simulink model "W01_Base_World_point_cloud_performance_cs"  (R2019a)
settings: Solver=FixedStepDiscrete  StartTime=0.0  StopTime=612  FixedStep=1/20  RelTol=1e-3
PreLoadFcn:
  | mbxruntime.callbacks.PreLoadFcn(bdroot);
  | check_NUTS_defined
  | model_closed = 0;
  | assignin('base',['model_closed_' bdroot],false);
PostLoadFcn:
  | mbxruntime.callbacks.PostLoadFcn(bdroot);
InitFcn:
  | mbxruntime.callbacks.InitFcn(bdroot);
StartFcn:
  | mbxruntime.callbacks.StartFcn(bdroot);
StopFcn:
  | mbxruntime.callbacks.StopFcn(bdroot);;
  | 
model workspace: external: MAT-File .\W01_Base_World_point_cloud_performance_cs_hws.mat (data not in the file)
undefined symbols (not defined in the file or in its folder): DiscIntNeverNeededParam, mbxruntime, Orientation, Position, tabledata, W01_Base_World_point_cloud_performance_cs_040d40f1a6998015, W01_Base_World_point_cloud_performance_cs_1139c7b998f0a907, W01_Base_World_point_cloud_performance_cs_282394bd9d11aaf9, W01_Base_World_point_cloud_performance_cs_287b60bdf29e1a5e, W01_Base_World_point_cloud_performance_cs_3d871abdbcb86cf3, W01_Base_World_point_cloud_performance_cs_8fcb18657fabefaa, W01_Base_World_point_cloud_performance_cs_9753c0e86959d2d1, W01_Base_World_point_cloud_performance_cs_9a36d3aa72057750, W01_Base_World_point_cloud_performance_cs_9a6e020116cabe98, W01_Base_World_point_cloud_performance_cs_a4ac4280946ec032, W01_Base_World_point_cloud_performance_cs_bbd2f0877d622aa1, W01_Base_World_point_cloud_performance_cs_d5d898f74cbe8316, W01_Base_World_point_cloud_performance_cs_d7d451946b8970f9, W01_Base_World_point_cloud_performance_cs_ed2f0fc632b9c889, W01_Base_World_point_cloud_performance_cs_f0849590441458e2, W01_Base_World_point_cloud_performance_cs_fc0d0ecba8ca3fae
libraries: simulink_extras x30, simulink x10, adeye_lib x6, sharedtransform x2, robotlib x2
(part 2 of 8)

== system W01_Base_World_point_cloud_performance_cs/ANIM_Child_RegularAni_1 ==
  ANIM_Child_RegularAni_1 : Inport  Tag=inport/AnimationOutport  OutDataTypeStr=Bus: PRESCAN_ANIMACTUATORDATA  PortDimensions=1  SampleTime=1/20  BusOutputAsStruct=on
  Actuator : S-Function  FunctionName=sfun_AnimActuator  Parameters=mbxruntime.parameters.convert(UniqueID), mbxruntime.parameters.convert(TimeStep)  SFunctionDeploymentMode=off  EnableBusSupport=off  mask(PreScan Sink Block: State Animation){UniqueID=18395, TimeStep=1/20}
      mask prompts: UniqueID "Auto-Assigned: Unique ID"; TimeStep "Auto-Assigned: Upload Period [s]"
      mask help: The Human Animation port allows the human to walk, run or bend
      mask Help: eval('openHelp(239)')
      mask Display: image(imread('HumanAnimated.jpg'))
  wires:
  ANIM_Child_RegularAni_1/1 -> Actuator/1

== system W01_Base_World_point_cloud_performance_cs/ANIM_Child_RegularAni_2 ==
  ANIM_Child_RegularAni_2 : Inport  Tag=inport/AnimationOutport  OutDataTypeStr=Bus: PRESCAN_ANIMACTUATORDATA  PortDimensions=1  SampleTime=1/20  BusOutputAsStruct=on
  Actuator : S-Function  FunctionName=sfun_AnimActuator  Parameters=mbxruntime.parameters.convert(UniqueID), mbxruntime.parameters.convert(TimeStep)  SFunctionDeploymentMode=off  EnableBusSupport=off  mask(PreScan Sink Block: State Animation){UniqueID=18628, TimeStep=1/20}
      mask prompts: UniqueID "Auto-Assigned: Unique ID"; TimeStep "Auto-Assigned: Upload Period [s]"
      mask help: The Human Animation port allows the human to walk, run or bend
      mask Help: eval('openHelp(239)')
      mask Display: image(imread('HumanAnimated.jpg'))
  wires:
  ANIM_Child_RegularAni_2/1 -> Actuator/1

== system W01_Base_World_point_cloud_performance_cs/ANIM_Female_RegularAni_1 ==
  ANIM_Female_RegularAni_1 : Inport  Tag=inport/AnimationOutport  OutDataTypeStr=Bus: PRESCAN_ANIMACTUATORDATA  PortDimensions=1  SampleTime=1/20  BusOutputAsStruct=on
  Actuator : S-Function  FunctionName=sfun_AnimActuator  Parameters=mbxruntime.parameters.convert(UniqueID), mbxruntime.parameters.convert(TimeStep)  SFunctionDeploymentMode=off  EnableBusSupport=off  mask(PreScan Sink Block: State Animation){UniqueID=18631, TimeStep=1/20}
      mask prompts: UniqueID "Auto-Assigned: Unique ID"; TimeStep "Auto-Assigned: Upload Period [s]"
      mask help: The Human Animation port allows the human to walk, run or bend
      mask Help: eval('openHelp(239)')
      mask Display: image(imread('HumanAnimated.jpg'))
  wires:
  ANIM_Female_RegularAni_1/1 -> Actuator/1

== system W01_Base_World_point_cloud_performance_cs/ANIM_Male_RegularAni_1 ==
  ANIM_Male_RegularAni_1 : Inport  Tag=inport/AnimationOutport  OutDataTypeStr=Bus: PRESCAN_ANIMACTUATORDATA  PortDimensions=1  SampleTime=1/20  BusOutputAsStruct=on
  Actuator : S-Function  FunctionName=sfun_AnimActuator  Parameters=mbxruntime.parameters.convert(UniqueID), mbxruntime.parameters.convert(TimeStep)  SFunctionDeploymentMode=off  EnableBusSupport=off  mask(PreScan Sink Block: State Animation){UniqueID=18634, TimeStep=1/20}
      mask prompts: UniqueID "Auto-Assigned: Unique ID"; TimeStep "Auto-Assigned: Upload Period [s]"
      mask help: The Human Animation port allows the human to walk, run or bend
      mask Help: eval('openHelp(239)')
      mask Display: image(imread('HumanAnimated.jpg'))
  wires:
  ANIM_Male_RegularAni_1/1 -> Actuator/1

== system W01_Base_World_point_cloud_performance_cs/ANIM_Male_RegularAni_2 ==
  ANIM_Male_RegularAni_2 : Inport  Tag=inport/AnimationOutport  OutDataTypeStr=Bus: PRESCAN_ANIMACTUATORDATA  PortDimensions=1  SampleTime=1/20  BusOutputAsStruct=on
  Actuator : S-Function  FunctionName=sfun_AnimActuator  Parameters=mbxruntime.parameters.convert(UniqueID), mbxruntime.parameters.convert(TimeStep)  SFunctionDeploymentMode=off  EnableBusSupport=off  mask(PreScan Sink Block: State Animation){UniqueID=18853, TimeStep=1/20}
      mask prompts: UniqueID "Auto-Assigned: Unique ID"; TimeStep "Auto-Assigned: Upload Period [s]"
      mask help: The Human Animation port allows the human to walk, run or bend
      mask Help: eval('openHelp(239)')
      mask Display: image(imread('HumanAnimated.jpg'))
  wires:
  ANIM_Male_RegularAni_2/1 -> Actuator/1

== system W01_Base_World_point_cloud_performance_cs/Audi_A8_Sedan_1 ==
  SELF_Audi_A8_Sedan_1 : Inport  Tag=inport/SelfPort  OutDataTypeStr=Bus: PRESCAN_SELFSENSORDATA  PortDimensions=1  SampleTime=1/20  BusOutputAsStruct=on
  Car_Pos_and_Orient : Subsystem
  Path : S-Function  LoadFcn=load('PrescanMotionData.mat')  FunctionName=sfun_Path  Parameters=mbxruntime.parameters.convert(uniqueID), pathUniqueID, mbxruntime.parameters.convert(timestep)  SFunctionDeploymentMode=off  EnableBusSupport=off  mask(Path){uniqueID=18645, pathUniqueID=W01_Base_World_point_cloud_performance_cs_f0849590441458e2, timestep=1/20}
      mask prompts: uniqueID "Object Unique ID"; pathUniqueID "Path Unique ID"; timestep "MATLAB timestep:"
      mask help:
      | The path block outputs the position along a given trajectory.
      |
      | For more information, please click Help.
      mask Help: eval('openHelp(312)')
      mask Display: image(imread('Path.png'))
  SELF_Demux : Subsystem  Tag=demux/SelfPort  mask(PreScan Demux Block:){}
      mask help:
      | The SELF port shows (state) information of the actor itself. The outputs are position in the experiment's axis system and the GPS coordinates, and the object's absolute velocity and compass heading.
      |
      | For more information, please click Help.
      settings: DeleteFcn=PreScanBlockDeleteFcn;
      mask Help: eval('openHelp(462)')
      mask Display:
      | port_label('output',1,'x [m]')
      | port_label('output',2,'y [m]')
      | port_label('output',3,'z [m]','texmode','on')
      | port_label('output',4,'Rotx [deg]','texmode','on')
      | port_label('output',5,'Roty [deg]','texmode','on')
      | port_label('output',6,'Rotz [deg]','texmode','on')
      | port_label('output',7,'GPS lat [deg]','texmode','on')
      | port_label('output',8,'GPS long [deg]','texmode','on')
      | port_label('output',9,'GPS alt [m]','texmode','on')
      | port_label('output',10,'Velocity [m/s]')
      | port_label('output',11,'Heading [deg]')
      | port_label('output',12,'Yaw rate [deg/s]')
      | port_label('output',13,'Timestamp [s]')
  STATE_Audi_A8_Sedan_1_rc : RateTransition  Tag=mux_rc/StatePort  OutPortSampleTimeOpt=Inherit
  SpeedProfile : S-Function  LoadFcn=load('PrescanMotionData.mat')  FunctionName=sfun_SpeedProfile  Parameters=speedProfileUniqueID, mbxruntime.parameters.convert(timestep)  SFunctionDeploymentMode=off  EnableBusSupport=off  mask(SpeedProfile){speedProfileUniqueID=W01_Base_World_point_cloud_performance_cs_a4ac4280946ec032, timestep=1/20}
      mask prompts: speedProfileUniqueID "Speed Profile Unique ID"; timestep "MATLAB timestep:"
      mask help:
      | The speed profile block outputs the travelled distance, velocities and acceleration along a given path.
      |
      | For more information, please click Help.
      mask Help: eval('openHelp(312)')
      mask Display: image(imread('SpeedProfile.png'))
  Terminator_{1..7} (7 alike) : Terminator
  message_creator : Subsystem
  STATE_Audi_A8_Sedan_1_bus : Outport  Tag=outport/StatePort  OutDataTypeStr=Bus: PRESCAN_STATEACTUATORDATA  PortDimensions=1  SampleTime=1/20
  SafetyPlannerLoc : Outport  Port=2
  wires:
  Car_Pos_and_Orient/1(Out1) -> message_creator/1(In1)
  message_creator/1(Out1) -> SafetyPlannerLoc/1
  SELF_Demux/1(x [m]) -> Car_Pos_and_Orient/1(In1)
  SELF_Demux/2(y [m]) -> Car_Pos_and_Orient/2(In2)
  SELF_Demux/3(z [m]) -> Car_Pos_and_Orient/3(In3)
  SELF_Demux/4(rotx [deg]) -> Car_Pos_and_Orient/4(In4)
  SELF_Demux/5(roty [deg]) -> Car_Pos_and_Orient/5(In5)
  SELF_Demux/6(rotz [deg]) -> Car_Pos_and_Orient/6(In6)
  STATE_Audi_A8_Sedan_1_rc/1 -> STATE_Audi_A8_Sedan_1_bus/1
  SpeedProfile/1 -> Path/1
  Path/1 -> STATE_Audi_A8_Sedan_1_rc/1
  SELF_Audi_A8_Sedan_1/1 -> SELF_Demux/1(SELF)
  SELF_Demux/7(GPS lat [deg]) -> Terminator_1/1
  SELF_Demux/8(GPS long [deg]) -> Terminator_2/1
  SELF_Demux/9(GPS alt [m]) -> Terminator_3/1
  SELF_Demux/10(velocity [m/s]) -> Terminator_4/1
  SELF_Demux/11(heading [deg]) -> Terminator_5/1
  SELF_Demux/12(yaw rate [deg/s]) -> Terminator_6/1
  SELF_Demux/13(TimeStamp [s]) -> Terminator_7/1

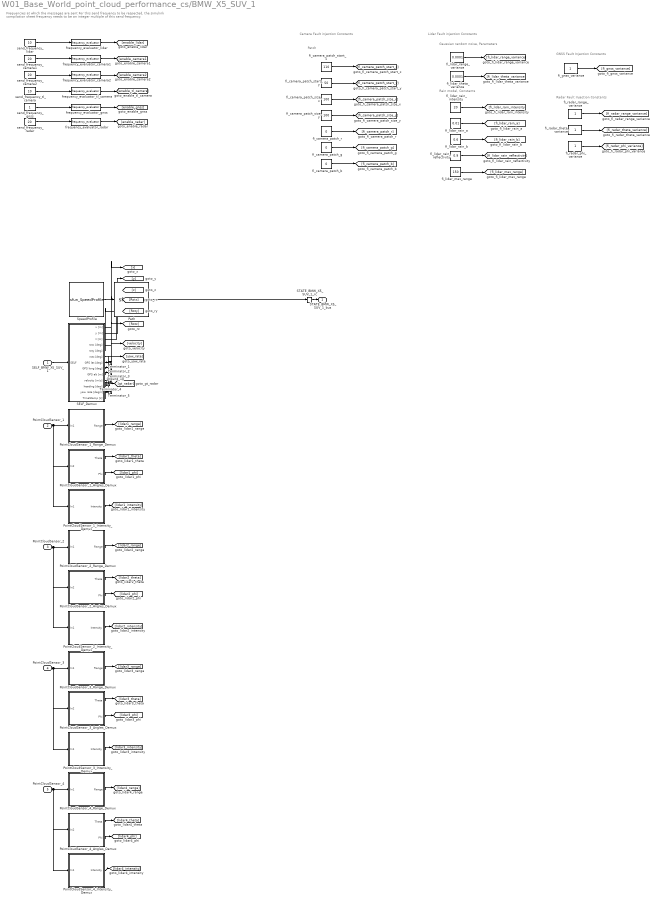
== system W01_Base_World_point_cloud_performance_cs/BMW_X5_SUV_1 ==
  note: Frequencies at which the messages are sent
      |
      | For this send frequency to be respected, the simulink compilation sheet frequency
      | needs to be an integer multiple of this send frequency.
  note: Lidar Fault injection Constants
  note: Camera Fault injection Constants
  note: Patch
  note: Rain model, Constants
  note: Radar Fault Injection Constants
  note: Gaussian random noise, Parameters
  note: GNSS Fault Injection Constants
  SELF_BMW_X5_SUV_1 : Inport  Tag=inport/SelfPort  OutDataTypeStr=Bus: PRESCAN_SELFSENSORDATA  PortDimensions=1  SampleTime=1/20  BusOutputAsStruct=on
  PointCloudSensor_1 : Inport  Tag=inport/PointCloudInport  Port=2  OutDataTypeStr=single  SampleTime=1/10  BusOutputAsStruct=on
  PointCloudSensor_2 : Inport  Tag=inport/PointCloudInport  Port=3  OutDataTypeStr=single  SampleTime=1/10  BusOutputAsStruct=on
  PointCloudSensor_3 : Inport  Tag=inport/PointCloudInport  Port=4  OutDataTypeStr=single  SampleTime=1/10  BusOutputAsStruct=on
  PointCloudSensor_4 : Inport  Tag=inport/PointCloudInport  Port=5  OutDataTypeStr=single  SampleTime=1/10  BusOutputAsStruct=on
  Ground_10 : Ground
  Path : S-Function  LoadFcn=load('PrescanMotionData.mat')  FunctionName=sfun_Path  Parameters=mbxruntime.parameters.convert(uniqueID), pathUniqueID, mbxruntime.parameters.convert(timestep)  SFunctionDeploymentMode=off  EnableBusSupport=off  mask(Path){uniqueID=9040, pathUniqueID=W01_Base_World_point_cloud_performance_cs_9a36d3aa72057750, timestep=1/20}
      mask prompts: uniqueID "Object Unique ID"; pathUniqueID "Path Unique ID"; timestep "MATLAB timestep:"
      mask help:
      | The path block outputs the position along a given trajectory.
      |
      | For more information, please click Help.
      mask Help: eval('openHelp(312)')
      mask Display: image(imread('Path.png'))
  PointCloudSensor_1_Angles_Demux : Subsystem  Tag=demux/PCS/Angles  mask{SensorName=PointCloudSensor_1, offset=225, hres=225, vres=16}
      mask prompts: SensorName "Sensor Name"; offset "Data Start"; hres "Horizontal Resolution"; vres "Vertical Resolution"
      mask Help: eval('openHelp(6400)')
      mask Display:
      | fprintf('Point Cloud:\n Data\n %s \n %d x %d px',SensorName,hres,vres)
      | port_label('output',1,'Theta')
      | port_label('output',2,'Phi')
  PointCloudSensor_1_Intensity_Demux : Subsystem  Tag=demux/PCS/Intensity  mask{SensorName=PointCloudSensor_1, offset=675, hres=225, vres=16}
      mask prompts: SensorName "Sensor Name"; offset "Data Start"; hres "Horizontal Resolution"; vres "Vertical Resolution"
      mask Help: eval('openHelp(6400)')
      mask Display:
      | fprintf('Point Cloud:\n Data\n %s \n %d x %d px',SensorName,hres,vres)
      | port_label('output',1,'Intensity')
  PointCloudSensor_1_Range_Demux : Subsystem  Tag=demux/PCS/Range  mask{SensorName=PointCloudSensor_1, offset=0, hres=225, vres=16}
      mask prompts: SensorName "Sensor Name"; offset "Data Start"; hres "Horizontal Resolution"; vres "Vertical Resolution"
      mask Help: eval('openHelp(6400)')
      mask Display:
      | fprintf('Point Cloud:\n Data\n %s \n %d x %d px',SensorName,hres,vres)
      | port_label('output',1,'Range')
  PointCloudSensor_2_Angles_Demux : Subsystem  Tag=demux/PCS/Angles  mask{SensorName=PointCloudSensor_2, offset=225, hres=225, vres=16}
      mask prompts: SensorName "Sensor Name"; offset "Data Start"; hres "Horizontal Resolution"; vres "Vertical Resolution"
      mask Help: eval('openHelp(6400)')
      mask Display:
      | fprintf('Point Cloud:\n Data\n %s \n %d x %d px',SensorName,hres,vres)
      | port_label('output',1,'Theta')
      | port_label('output',2,'Phi')
  PointCloudSensor_2_Intensity_Demux : Subsystem  Tag=demux/PCS/Intensity  mask{SensorName=PointCloudSensor_2, offset=675, hres=225, vres=16}
      mask prompts: SensorName "Sensor Name"; offset "Data Start"; hres "Horizontal Resolution"; vres "Vertical Resolution"
      mask Help: eval('openHelp(6400)')
      mask Display:
      | fprintf('Point Cloud:\n Data\n %s \n %d x %d px',SensorName,hres,vres)
      | port_label('output',1,'Intensity')
  PointCloudSensor_2_Range_Demux : Subsystem  Tag=demux/PCS/Range  mask{SensorName=PointCloudSensor_2, offset=0, hres=225, vres=16}
      mask prompts: SensorName "Sensor Name"; offset "Data Start"; hres "Horizontal Resolution"; vres "Vertical Resolution"
      mask Help: eval('openHelp(6400)')
      mask Display:
      | fprintf('Point Cloud:\n Data\n %s \n %d x %d px',SensorName,hres,vres)
      | port_label('output',1,'Range')
  PointCloudSensor_3_Angles_Demux : Subsystem  Tag=demux/PCS/Angles  mask{SensorName=PointCloudSensor_3, offset=225, hres=225, vres=16}
      mask prompts: SensorName "Sensor Name"; offset "Data Start"; hres "Horizontal Resolution"; vres "Vertical Resolution"
      mask Help: eval('openHelp(6400)')
      mask Display:
      | fprintf('Point Cloud:\n Data\n %s \n %d x %d px',SensorName,hres,vres)
      | port_label('output',1,'Theta')
      | port_label('output',2,'Phi')
  PointCloudSensor_3_Intensity_Demux : Subsystem  Tag=demux/PCS/Intensity  mask{SensorName=PointCloudSensor_3, offset=675, hres=225, vres=16}
      mask prompts: SensorName "Sensor Name"; offset "Data Start"; hres "Horizontal Resolution"; vres "Vertical Resolution"
      mask Help: eval('openHelp(6400)')
      mask Display:
      | fprintf('Point Cloud:\n Data\n %s \n %d x %d px',SensorName,hres,vres)
      | port_label('output',1,'Intensity')
  PointCloudSensor_3_Range_Demux : Subsystem  Tag=demux/PCS/Range  mask{SensorName=PointCloudSensor_3, offset=0, hres=225, vres=16}
      mask prompts: SensorName "Sensor Name"; offset "Data Start"; hres "Horizontal Resolution"; vres "Vertical Resolution"
      mask Help: eval('openHelp(6400)')
      mask Display:
      | fprintf('Point Cloud:\n Data\n %s \n %d x %d px',SensorName,hres,vres)
      | port_label('output',1,'Range')
  PointCloudSensor_4_Angles_Demux : Subsystem  Tag=demux/PCS/Angles  mask{SensorName=PointCloudSensor_4, offset=225, hres=225, vres=16}
      mask prompts: SensorName "Sensor Name"; offset "Data Start"; hres "Horizontal Resolution"; vres "Vertical Resolution"
      mask Help: eval('openHelp(6400)')
      mask Display:
      | fprintf('Point Cloud:\n Data\n %s \n %d x %d px',SensorName,hres,vres)
      | port_label('output',1,'Theta')
      | port_label('output',2,'Phi')
  PointCloudSensor_4_Intensity_Demux : Subsystem  Tag=demux/PCS/Intensity  mask{SensorName=PointCloudSensor_4, offset=675, hres=225, vres=16}
      mask prompts: SensorName "Sensor Name"; offset "Data Start"; hres "Horizontal Resolution"; vres "Vertical Resolution"
      mask Help: eval('openHelp(6400)')
      mask Display:
      | fprintf('Point Cloud:\n Data\n %s \n %d x %d px',SensorName,hres,vres)
      | port_label('output',1,'Intensity')
  PointCloudSensor_4_Range_Demux : Subsystem  Tag=demux/PCS/Range  mask{SensorName=PointCloudSensor_4, offset=0, hres=225, vres=16}
      mask prompts: SensorName "Sensor Name"; offset "Data Start"; hres "Horizontal Resolution"; vres "Vertical Resolution"
      mask Help: eval('openHelp(6400)')
      mask Display:
      | fprintf('Point Cloud:\n Data\n %s \n %d x %d px',SensorName,hres,vres)
      | port_label('output',1,'Range')
  SELF_Demux : Subsystem  Tag=demux/SelfPort  mask(PreScan Demux Block:){}
      mask help:
      | The SELF port shows (state) information of the actor itself. The outputs are position in the experiment's axis system and the GPS coordinates, and the object's absolute velocity and compass heading.
      |
      | For more information, please click Help.
      settings: DeleteFcn=PreScanBlockDeleteFcn;
      mask Help: eval('openHelp(462)')
      mask Display:
      | port_label('output',1,'x [m]')
      | port_label('output',2,'y [m]')
      | port_label('output',3,'z [m]','texmode','on')
      | port_label('output',4,'Rotx [deg]','texmode','on')
      | port_label('output',5,'Roty [deg]','texmode','on')
      | port_label('output',6,'Rotz [deg]','texmode','on')
      | port_label('output',7,'GPS lat [deg]','texmode','on')
      | port_label('output',8,'GPS long [deg]','texmode','on')
      | port_label('output',9,'GPS alt [m]','texmode','on')
      | port_label('output',10,'Velocity [m/s]')
      | port_label('output',11,'Heading [deg]')
      | port_label('output',12,'Yaw rate [deg/s]')
      | port_label('output',13,'Timestamp [s]')
  STATE_BMW_X5_SUV_1_rc : RateTransition  Tag=mux_rc/StatePort  OutPortSampleTimeOpt=Inherit
  SpeedProfile : S-Function  LoadFcn=load('PrescanMotionData.mat')  FunctionName=sfun_SpeedProfile  Parameters=speedProfileUniqueID, mbxruntime.parameters.convert(timestep)  SFunctionDeploymentMode=off  EnableBusSupport=off  mask(SpeedProfile){speedProfileUniqueID=W01_Base_World_point_cloud_performance_cs_9753c0e86959d2d1, timestep=1/20}
      mask prompts: speedProfileUniqueID "Speed Profile Unique ID"; timestep "MATLAB timestep:"
      mask help:
      | The speed profile block outputs the travelled distance, velocities and acceleration along a given path.
      |
      | For more information, please click Help.
      mask Help: eval('openHelp(312)')
      mask Display: image(imread('SpeedProfile.png'))
  Terminator_{1..5} (5 alike) : Terminator
  fi_camera_patch_b : Constant  Value=0
  fi_camera_patch_g : Constant  Value=0
  fi_camera_patch_r : Constant  Value=0
  fi_camera_patch_size_x : Constant  Value=100
  fi_camera_patch_size_y : Constant  Value=100
  fi_camera_patch_start_x : Constant  Value=110
  fi_camera_patch_start_y : Constant  Value=50
  fi_gnss_variance : Constant
  fi_lidar_max_range : Constant  Value=150
  fi_lidar_rain_a : Constant  Value=0.01
  fi_lidar_rain_b : Constant  Value=0.6
  fi_lidar_rain_intensity : Constant  Value=20
  fi_lidar_rain_reflectivity : Constant  Value=0.9
  fi_lidar_range_variance : Constant  Value=0.0001
  fi_lidar_theta_variance : Constant  Value=0.0001
  fi_radar_phi_variance : Constant
  fi_radar_range_variance : Constant
  fi_radar_theta_variance : Constant
  frequency_evaluator_camera1 : adeye_lib/frequency_evaluator  SystemSampleTime=-1
  frequency_evaluator_camera2 : adeye_lib/frequency_evaluator  SystemSampleTime=-1
  frequency_evaluator_gnss : adeye_lib/frequency_evaluator  SystemSampleTime=-1
  frequency_evaluator_lidar : adeye_lib/frequency_evaluator  SystemSampleTime=-1
      link override Constant: Value=0.999
  frequency_evaluator_radar : adeye_lib/frequency_evaluator  SystemSampleTime=-1
  frequency_evaluator_tl_camera : adeye_lib/frequency_evaluator  SystemSampleTime=-1
  send_frequency_camera1 : Constant  Value=20
  send_frequency_camera2 : Constant  Value=20
  send_frequency_gnss : Constant
  send_frequency_lidar : Constant  Value=10
  send_frequency_radar : Constant  Value=20
  send_frequency_tl_camera : Constant  Value=10
  STATE_BMW_X5_SUV_1_bus : Outport  Tag=outport/StatePort  OutDataTypeStr=Bus: PRESCAN_STATEACTUATORDATA  PortDimensions=1  SampleTime=1/20
  wires:
  fi_camera_patch_b/1 -> [fi_camera_patch_b]
  fi_camera_patch_g/1 -> [fi_camera_patch_g]
  fi_camera_patch_r/1 -> [fi_camera_patch_r]
  fi_camera_patch_size_x/1 -> [fi_camera_patch_size_x]
  fi_camera_patch_size_y/1 -> [fi_camera_patch_size_y]
  fi_camera_patch_start_x/1 -> [fi_camera_patch_start_x]
  fi_camera_patch_start_y/1 -> [fi_camera_patch_start_y]
  fi_gnss_variance/1 -> [fi_gnss_variance]
  fi_lidar_max_range/1 -> [fi_lidar_max_range]
  fi_lidar_rain_a/1 -> [fi_lidar_rain_a]
  fi_lidar_rain_b/1 -> [fi_lidar_rain_b]
  fi_lidar_rain_intensity/1 -> [fi_lidar_rain_intensity]
  fi_lidar_rain_reflectivity/1 -> [fi_lidar_rain_reflectivity]
  fi_lidar_range_variance/1 -> [fi_lidar_range_variance]
  fi_lidar_theta_variance/1 -> [fi_lidar_theta_variance]
  fi_radar_phi_variance/1 -> [fi_radar_phi_variance]
  fi_radar_range_variance/1 -> [fi_radar_range_variance]
  fi_radar_theta_variance/1 -> [fi_radar_theta_variance]
  PointCloudSensor_1_Intensity_Demux/1(Intensity) -> [lidar1_intensity]
  PointCloudSensor_1_Angles_Demux/2(Phi) -> [lidar1_phi]
  PointCloudSensor_1_Range_Demux/1(Range) -> [lidar1_range]
  PointCloudSensor_1_Angles_Demux/1(Theta) -> [lidar1_theta]
  PointCloudSensor_2_Intensity_Demux/1(Intensity) -> [lidar2_intensity]
  PointCloudSensor_2_Angles_Demux/2(Phi) -> [lidar2_phi]
  PointCloudSensor_2_Range_Demux/1(Range) -> [lidar2_range]
  PointCloudSensor_2_Angles_Demux/1(Theta) -> [lidar2_theta]
  PointCloudSensor_3_Intensity_Demux/1(Intensity) -> [lidar3_intensity]
  PointCloudSensor_3_Angles_Demux/2(Phi) -> [lidar3_phi]
  PointCloudSensor_3_Range_Demux/1(Range) -> [lidar3_range]
  PointCloudSensor_3_Angles_Demux/1(Theta) -> [lidar3_theta]
  PointCloudSensor_4_Intensity_Demux/1(Intensity) -> [lidar4_intensity]
  PointCloudSensor_4_Angles_Demux/2(Phi) -> [lidar4_phi]
  PointCloudSensor_4_Range_Demux/1(Range) -> [lidar4_range]
  PointCloudSensor_4_Angles_Demux/1(Theta) -> [lidar4_theta]
  SELF_Demux/4(rotx [deg]) -> [Rotx]
  SELF_Demux/5(roty [deg]) -> [Roty]
  SELF_Demux/6(rotz [deg]) -> [Rotz]
  SELF_Demux/10(velocity [m/s]) -> [velocity]
  SELF_Demux/1(x [m]) -> [x]
  SELF_Demux/2(y [m]) -> [y]
  SELF_Demux/12(yaw rate [deg/s]) -> [yaw_rate]
  SELF_Demux/3(z [m]) -> [z]
  send_frequency_lidar/1 -> frequency_evaluator_lidar/1
  send_frequency_camera1/1 -> frequency_evaluator_camera1/1
  send_frequency_camera2/1 -> frequency_evaluator_camera2/1
  send_frequency_tl_camera/1 -> frequency_evaluator_tl_camera/1
  send_frequency_gnss/1 -> frequency_evaluator_gnss/1
  frequency_evaluator_lidar/1 -> [enable_lidar]
  frequency_evaluator_camera1/1 -> [enable_camera1]
  frequency_evaluator_camera2/1 -> [enable_camera2]
  frequency_evaluator_tl_camera/1 -> [enable_tl_camera]
  frequency_evaluator_gnss/1 -> [enable_gnss]
  send_frequency_radar/1 -> frequency_evaluator_radar/1
  frequency_evaluator_radar/1 -> [enable_radar]
  STATE_BMW_X5_SUV_1_rc/1 -> STATE_BMW_X5_SUV_1_bus/1
  SpeedProfile/1 -> Path/1
  Path/1 -> STATE_BMW_X5_SUV_1_rc/1
  SELF_BMW_X5_SUV_1/1 -> SELF_Demux/1(SELF)
  PointCloudSensor_1/1 -> PointCloudSensor_1_Range_Demux/1(In1), PointCloudSensor_1_Angles_Demux/1(In2), PointCloudSensor_1_Intensity_Demux/1(In1)
  PointCloudSensor_2/1 -> PointCloudSensor_2_Range_Demux/1(In1), PointCloudSensor_2_Angles_Demux/1(In2), PointCloudSensor_2_Intensity_Demux/1(In1)
  PointCloudSensor_3/1 -> PointCloudSensor_3_Range_Demux/1(In1), PointCloudSensor_3_Angles_Demux/1(In2), PointCloudSensor_3_Intensity_Demux/1(In1)
  PointCloudSensor_4/1 -> PointCloudSensor_4_Range_Demux/1(In1), PointCloudSensor_4_Angles_Demux/1(In2), PointCloudSensor_4_Intensity_Demux/1(In1)
  SELF_Demux/7(GPS lat [deg]) -> Terminator_1/1
  SELF_Demux/8(GPS long [deg]) -> Terminator_2/1
  SELF_Demux/9(GPS alt [m]) -> Terminator_3/1
  SELF_Demux/11(heading [deg]) -> Terminator_4/1
  SELF_Demux/13(TimeStamp [s]) -> Terminator_5/1
  Ground_10/1 -> [gt_radar]

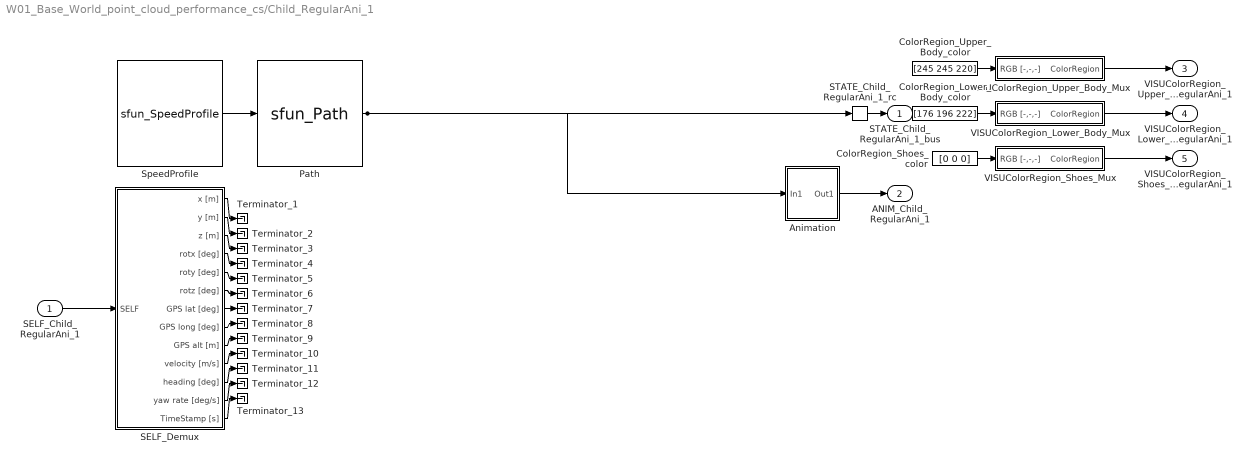
== system W01_Base_World_point_cloud_performance_cs/Child_RegularAni_1 ==
  SELF_Child_RegularAni_1 : Inport  Tag=inport/SelfPort  OutDataTypeStr=Bus: PRESCAN_SELFSENSORDATA  PortDimensions=1  SampleTime=1/20  BusOutputAsStruct=on
  Animation : Subsystem  Tag=RunningHumanAnimation  mask(Prescan Conversion Block: Running Human Animation){MWS=1.95, WalkingScale=1.0, RunningScale=1.0, TimeStep=1/20}
      mask prompts: MWS "Maximum Walking Speed [m/s], above which the animation will switch to running mode."; WalkingScale "Walking mode scaling factor to sync the animation frames to the displacement."; RunningScale "Running mode scaling factor to sync the animation frames to the displacement."; TimeStep "Auto-Assigned: Upload Period [s]"
      mask help: The Running Human Animation block converts the State signal of a human into signals to properly control the animation.
      mask Help: eval('openHelp(239)');
      mask Display: image(imread('HumanAnimated.jpg'))
  ColorRegion_Lower_Body_color : Constant  Tag=VisuLightConst  Value=[176 196 222]
  ColorRegion_Shoes_color : Constant  Tag=VisuLightConst  Value=[0 0 0]
  ColorRegion_Upper_Body_color : Constant  Tag=VisuLightConst  Value=[245 245 220]
  Path : S-Function  LoadFcn=load('PrescanMotionData.mat')  FunctionName=sfun_Path  Parameters=mbxruntime.parameters.convert(uniqueID), pathUniqueID, mbxruntime.parameters.convert(timestep)  SFunctionDeploymentMode=off  EnableBusSupport=off  mask(Path){uniqueID=18395, pathUniqueID=W01_Base_World_point_cloud_performance_cs_d7d451946b8970f9, timestep=1/20}
      mask prompts: uniqueID "Object Unique ID"; pathUniqueID "Path Unique ID"; timestep "MATLAB timestep:"
      mask help:
      | The path block outputs the position along a given trajectory.
      |
      | For more information, please click Help.
      mask Help: eval('openHelp(312)')
      mask Display: image(imread('Path.png'))
  SELF_Demux : Subsystem  Tag=demux/SelfPort  mask(PreScan Demux Block:){}
      mask help:
      | The SELF port shows (state) information of the actor itself. The outputs are position in the experiment's axis system and the GPS coordinates, and the object's absolute velocity and compass heading.
      |
      | For more information, please click Help.
      settings: DeleteFcn=PreScanBlockDeleteFcn;
      mask Help: eval('openHelp(462)')
      mask Display:
      | port_label('output',1,'x [m]')
      | port_label('output',2,'y [m]')
      | port_label('output',3,'z [m]','texmode','on')
      | port_label('output',4,'Rotx [deg]','texmode','on')
      | port_label('output',5,'Roty [deg]','texmode','on')
      | port_label('output',6,'Rotz [deg]','texmode','on')
      | port_label('output',7,'GPS lat [deg]','texmode','on')
      | port_label('output',8,'GPS long [deg]','texmode','on')
      | port_label('output',9,'GPS alt [m]','texmode','on')
      | port_label('output',10,'Velocity [m/s]')
      | port_label('output',11,'Heading [deg]')
      | port_label('output',12,'Yaw rate [deg/s]')
      | port_label('output',13,'Timestamp [s]')
  STATE_Child_RegularAni_1_rc : RateTransition  Tag=mux_rc/StatePort  OutPortSampleTimeOpt=Inherit
  SpeedProfile : S-Function  LoadFcn=load('PrescanMotionData.mat')  FunctionName=sfun_SpeedProfile  Parameters=speedProfileUniqueID, mbxruntime.parameters.convert(timestep)  SFunctionDeploymentMode=off  EnableBusSupport=off  mask(SpeedProfile){speedProfileUniqueID=W01_Base_World_point_cloud_performance_cs_bbd2f0877d622aa1, timestep=1/20}
      mask prompts: speedProfileUniqueID "Speed Profile Unique ID"; timestep "MATLAB timestep:"
      mask help:
      | The speed profile block outputs the travelled distance, velocities and acceleration along a given path.
      |
      | For more information, please click Help.
      mask Help: eval('openHelp(312)')
      mask Display: image(imread('SpeedProfile.png'))
  Terminator_{1..13} (13 alike) : Terminator
  VISUColorRegion_Lower_Body_Mux : Subsystem  Tag=mux/MuxColorRegion  LoadFcn=load PrescanColorData  mask(PreScan User Interface: VisuTextureColor){}
      mask help:
      | The VisuTextureColor block provides a way to adapt the color of a vehicle.
      |
      | For more information, please click Help.
      settings: DeleteFcn=PreScanBlockDeleteFcn;
      mask Help: eval('openHelp(230)')
  VISUColorRegion_Shoes_Mux : Subsystem  Tag=mux/MuxColorRegion  LoadFcn=load PrescanColorData  mask(PreScan User Interface: VisuTextureColor){}
      mask help:
      | The VisuTextureColor block provides a way to adapt the color of a vehicle.
      |
      | For more information, please click Help.
      settings: DeleteFcn=PreScanBlockDeleteFcn;
      mask Help: eval('openHelp(230)')
  VISUColorRegion_Upper_Body_Mux : Subsystem  Tag=mux/MuxColorRegion  LoadFcn=load PrescanColorData  mask(PreScan User Interface: VisuTextureColor){}
      mask help:
      | The VisuTextureColor block provides a way to adapt the color of a vehicle.
      |
      | For more information, please click Help.
      settings: DeleteFcn=PreScanBlockDeleteFcn;
      mask Help: eval('openHelp(230)')
  STATE_Child_RegularAni_1_bus : Outport  Tag=outport/StatePort  OutDataTypeStr=Bus: PRESCAN_STATEACTUATORDATA  PortDimensions=1  SampleTime=1/20
  ANIM_Child_RegularAni_1 : Outport  Tag=outport/AnimationOutport  Port=2  OutDataTypeStr=Bus: PRESCAN_ANIMACTUATORDATA  PortDimensions=1  SampleTime=1/20
  VISUColorRegion_Upper_Body_Child_RegularAni_1 : Outport  Tag=outport/ColorRegion  Port=3  OutDataTypeStr=Bus: PRESCAN_COLOR_DATA  PortDimensions=1  SampleTime=1/20
  VISUColorRegion_Lower_Body_Child_RegularAni_1 : Outport  Tag=outport/ColorRegion  Port=4  OutDataTypeStr=Bus: PRESCAN_COLOR_DATA  PortDimensions=1  SampleTime=1/20
  VISUColorRegion_Shoes_Child_RegularAni_1 : Outport  Tag=outport/ColorRegion  Port=5  OutDataTypeStr=Bus: PRESCAN_COLOR_DATA  PortDimensions=1  SampleTime=1/20
  wires:
  STATE_Child_RegularAni_1_rc/1 -> STATE_Child_RegularAni_1_bus/1
  Animation/1(Out1) -> ANIM_Child_RegularAni_1/1
  SpeedProfile/1 -> Path/1
  Path/1 -> STATE_Child_RegularAni_1_rc/1, Animation/1(In1)
  SELF_Child_RegularAni_1/1 -> SELF_Demux/1(SELF)
  VISUColorRegion_Upper_Body_Mux/1(ColorRegion) -> VISUColorRegion_Upper_Body_Child_RegularAni_1/1
  ColorRegion_Upper_Body_color/1 -> VISUColorRegion_Upper_Body_Mux/1(RGB [-,-,-])
  VISUColorRegion_Lower_Body_Mux/1(ColorRegion) -> VISUColorRegion_Lower_Body_Child_RegularAni_1/1
  ColorRegion_Lower_Body_color/1 -> VISUColorRegion_Lower_Body_Mux/1(RGB [-,-,-])
  VISUColorRegion_Shoes_Mux/1(ColorRegion) -> VISUColorRegion_Shoes_Child_RegularAni_1/1
  ColorRegion_Shoes_color/1 -> VISUColorRegion_Shoes_Mux/1(RGB [-,-,-])
  SELF_Demux/1(x [m]) -> Terminator_1/1
  SELF_Demux/2(y [m]) -> Terminator_2/1
  SELF_Demux/3(z [m]) -> Terminator_3/1
  SELF_Demux/4(rotx [deg]) -> Terminator_4/1
  SELF_Demux/5(roty [deg]) -> Terminator_5/1
  SELF_Demux/6(rotz [deg]) -> Terminator_6/1
  SELF_Demux/7(GPS lat [deg]) -> Terminator_7/1
  SELF_Demux/8(GPS long [deg]) -> Terminator_8/1
  SELF_Demux/9(GPS alt [m]) -> Terminator_9/1
  SELF_Demux/10(velocity [m/s]) -> Terminator_10/1
  SELF_Demux/11(heading [deg]) -> Terminator_11/1
  SELF_Demux/12(yaw rate [deg/s]) -> Terminator_12/1
  SELF_Demux/13(TimeStamp [s]) -> Terminator_13/1

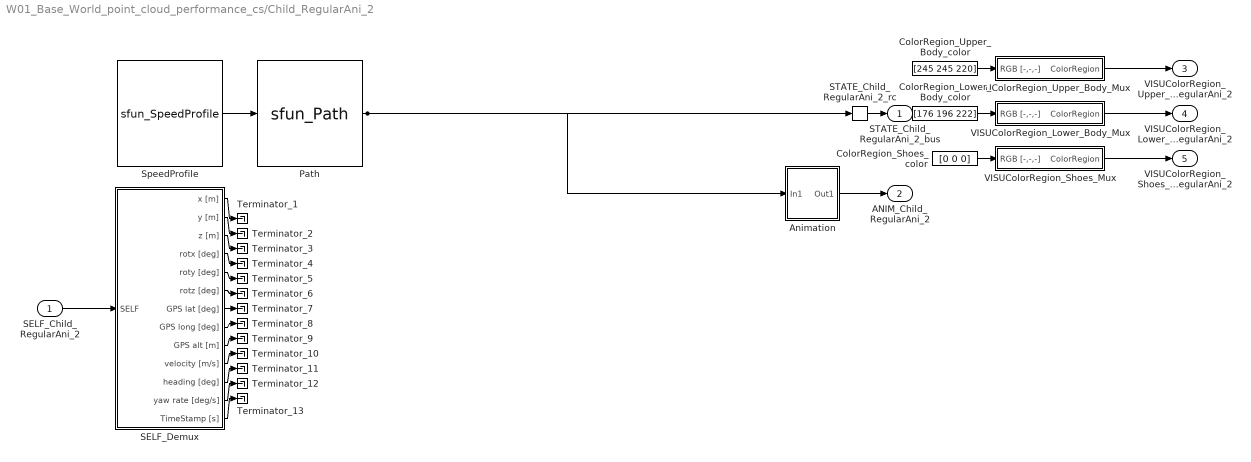
== system W01_Base_World_point_cloud_performance_cs/Child_RegularAni_2 ==
  SELF_Child_RegularAni_2 : Inport  Tag=inport/SelfPort  OutDataTypeStr=Bus: PRESCAN_SELFSENSORDATA  PortDimensions=1  SampleTime=1/20  BusOutputAsStruct=on
  Animation : Subsystem  Tag=RunningHumanAnimation  mask(Prescan Conversion Block: Running Human Animation){MWS=1.95, WalkingScale=1.0, RunningScale=1.0, TimeStep=1/20}
      mask prompts: MWS "Maximum Walking Speed [m/s], above which the animation will switch to running mode."; WalkingScale "Walking mode scaling factor to sync the animation frames to the displacement."; RunningScale "Running mode scaling factor to sync the animation frames to the displacement."; TimeStep "Auto-Assigned: Upload Period [s]"
      mask help: The Running Human Animation block converts the State signal of a human into signals to properly control the animation.
      mask Help: eval('openHelp(239)');
      mask Display: image(imread('HumanAnimated.jpg'))
  ColorRegion_Lower_Body_color : Constant  Tag=VisuLightConst  Value=[176 196 222]
  ColorRegion_Shoes_color : Constant  Tag=VisuLightConst  Value=[0 0 0]
  ColorRegion_Upper_Body_color : Constant  Tag=VisuLightConst  Value=[245 245 220]
  Path : S-Function  LoadFcn=load('PrescanMotionData.mat')  FunctionName=sfun_Path  Parameters=mbxruntime.parameters.convert(uniqueID), pathUniqueID, mbxruntime.parameters.convert(timestep)  SFunctionDeploymentMode=off  EnableBusSupport=off  mask(Path){uniqueID=18628, pathUniqueID=W01_Base_World_point_cloud_performance_cs_d5d898f74cbe8316, timestep=1/20}
      mask prompts: uniqueID "Object Unique ID"; pathUniqueID "Path Unique ID"; timestep "MATLAB timestep:"
      mask help:
      | The path block outputs the position along a given trajectory.
      |
      | For more information, please click Help.
      mask Help: eval('openHelp(312)')
      mask Display: image(imread('Path.png'))
  SELF_Demux : Subsystem  Tag=demux/SelfPort  mask(PreScan Demux Block:){}
      mask help:
      | The SELF port shows (state) information of the actor itself. The outputs are position in the experiment's axis system and the GPS coordinates, and the object's absolute velocity and compass heading.
      |
      | For more information, please click Help.
      settings: DeleteFcn=PreScanBlockDeleteFcn;
      mask Help: eval('openHelp(462)')
      mask Display:
      | port_label('output',1,'x [m]')
      | port_label('output',2,'y [m]')
      | port_label('output',3,'z [m]','texmode','on')
      | port_label('output',4,'Rotx [deg]','texmode','on')
      | port_label('output',5,'Roty [deg]','texmode','on')
      | port_label('output',6,'Rotz [deg]','texmode','on')
      | port_label('output',7,'GPS lat [deg]','texmode','on')
      | port_label('output',8,'GPS long [deg]','texmode','on')
      | port_label('output',9,'GPS alt [m]','texmode','on')
      | port_label('output',10,'Velocity [m/s]')
      | port_label('output',11,'Heading [deg]')
      | port_label('output',12,'Yaw rate [deg/s]')
      | port_label('output',13,'Timestamp [s]')
  STATE_Child_RegularAni_2_rc : RateTransition  Tag=mux_rc/StatePort  OutPortSampleTimeOpt=Inherit
  SpeedProfile : S-Function  LoadFcn=load('PrescanMotionData.mat')  FunctionName=sfun_SpeedProfile  Parameters=speedProfileUniqueID, mbxruntime.parameters.convert(timestep)  SFunctionDeploymentMode=off  EnableBusSupport=off  mask(SpeedProfile){speedProfileUniqueID=W01_Base_World_point_cloud_performance_cs_040d40f1a6998015, timestep=1/20}
      mask prompts: speedProfileUniqueID "Speed Profile Unique ID"; timestep "MATLAB timestep:"
      mask help:
      | The speed profile block outputs the travelled distance, velocities and acceleration along a given path.
      |
      | For more information, please click Help.
      mask Help: eval('openHelp(312)')
      mask Display: image(imread('SpeedProfile.png'))
  Terminator_{1..13} (13 alike) : Terminator
  VISUColorRegion_Lower_Body_Mux : Subsystem  Tag=mux/MuxColorRegion  LoadFcn=load PrescanColorData  mask(PreScan User Interface: VisuTextureColor){}
      mask help:
      | The VisuTextureColor block provides a way to adapt the color of a vehicle.
      |
      | For more information, please click Help.
      settings: DeleteFcn=PreScanBlockDeleteFcn;
      mask Help: eval('openHelp(230)')
  VISUColorRegion_Shoes_Mux : Subsystem  Tag=mux/MuxColorRegion  LoadFcn=load PrescanColorData  mask(PreScan User Interface: VisuTextureColor){}
      mask help:
      | The VisuTextureColor block provides a way to adapt the color of a vehicle.
      |
      | For more information, please click Help.
      settings: DeleteFcn=PreScanBlockDeleteFcn;
      mask Help: eval('openHelp(230)')
  VISUColorRegion_Upper_Body_Mux : Subsystem  Tag=mux/MuxColorRegion  LoadFcn=load PrescanColorData  mask(PreScan User Interface: VisuTextureColor){}
      mask help:
      | The VisuTextureColor block provides a way to adapt the color of a vehicle.
      |
      | For more information, please click Help.
      settings: DeleteFcn=PreScanBlockDeleteFcn;
      mask Help: eval('openHelp(230)')
  STATE_Child_RegularAni_2_bus : Outport  Tag=outport/StatePort  OutDataTypeStr=Bus: PRESCAN_STATEACTUATORDATA  PortDimensions=1  SampleTime=1/20
  ANIM_Child_RegularAni_2 : Outport  Tag=outport/AnimationOutport  Port=2  OutDataTypeStr=Bus: PRESCAN_ANIMACTUATORDATA  PortDimensions=1  SampleTime=1/20
  VISUColorRegion_Upper_Body_Child_RegularAni_2 : Outport  Tag=outport/ColorRegion  Port=3  OutDataTypeStr=Bus: PRESCAN_COLOR_DATA  PortDimensions=1  SampleTime=1/20
  VISUColorRegion_Lower_Body_Child_RegularAni_2 : Outport  Tag=outport/ColorRegion  Port=4  OutDataTypeStr=Bus: PRESCAN_COLOR_DATA  PortDimensions=1  SampleTime=1/20
  VISUColorRegion_Shoes_Child_RegularAni_2 : Outport  Tag=outport/ColorRegion  Port=5  OutDataTypeStr=Bus: PRESCAN_COLOR_DATA  PortDimensions=1  SampleTime=1/20
  wires:
  STATE_Child_RegularAni_2_rc/1 -> STATE_Child_RegularAni_2_bus/1
  Animation/1(Out1) -> ANIM_Child_RegularAni_2/1
  SpeedProfile/1 -> Path/1
  Path/1 -> STATE_Child_RegularAni_2_rc/1, Animation/1(In1)
  SELF_Child_RegularAni_2/1 -> SELF_Demux/1(SELF)
  VISUColorRegion_Upper_Body_Mux/1(ColorRegion) -> VISUColorRegion_Upper_Body_Child_RegularAni_2/1
  ColorRegion_Upper_Body_color/1 -> VISUColorRegion_Upper_Body_Mux/1(RGB [-,-,-])
  VISUColorRegion_Lower_Body_Mux/1(ColorRegion) -> VISUColorRegion_Lower_Body_Child_RegularAni_2/1
  ColorRegion_Lower_Body_color/1 -> VISUColorRegion_Lower_Body_Mux/1(RGB [-,-,-])
  VISUColorRegion_Shoes_Mux/1(ColorRegion) -> VISUColorRegion_Shoes_Child_RegularAni_2/1
  ColorRegion_Shoes_color/1 -> VISUColorRegion_Shoes_Mux/1(RGB [-,-,-])
  SELF_Demux/1(x [m]) -> Terminator_1/1
  SELF_Demux/2(y [m]) -> Terminator_2/1
  SELF_Demux/3(z [m]) -> Terminator_3/1
  SELF_Demux/4(rotx [deg]) -> Terminator_4/1
  SELF_Demux/5(roty [deg]) -> Terminator_5/1
  SELF_Demux/6(rotz [deg]) -> Terminator_6/1
  SELF_Demux/7(GPS lat [deg]) -> Terminator_7/1
  SELF_Demux/8(GPS long [deg]) -> Terminator_8/1
  SELF_Demux/9(GPS alt [m]) -> Terminator_9/1
  SELF_Demux/10(velocity [m/s]) -> Terminator_10/1
  SELF_Demux/11(heading [deg]) -> Terminator_11/1
  SELF_Demux/12(yaw rate [deg/s]) -> Terminator_12/1
  SELF_Demux/13(TimeStamp [s]) -> Terminator_13/1

== system W01_Base_World_point_cloud_performance_cs/Citroen_C3_Hatchback_1 ==
  SELF_Citroen_C3_Hatchback_1 : Inport  Tag=inport/SelfPort  OutDataTypeStr=Bus: PRESCAN_SELFSENSORDATA  PortDimensions=1  SampleTime=1/20  BusOutputAsStruct=on
  Car_Pos_and_Orient : Subsystem
  Path : S-Function  LoadFcn=load('PrescanMotionData.mat')  FunctionName=sfun_Path  Parameters=mbxruntime.parameters.convert(uniqueID), pathUniqueID, mbxruntime.parameters.convert(timestep)  SFunctionDeploymentMode=off  EnableBusSupport=off  mask(Path){uniqueID=18857, pathUniqueID=W01_Base_World_point_cloud_performance_cs_282394bd9d11aaf9, timestep=1/20}
      mask prompts: uniqueID "Object Unique ID"; pathUniqueID "Path Unique ID"; timestep "MATLAB timestep:"
      mask help:
      | The path block outputs the position along a given trajectory.
      |
      | For more information, please click Help.
      mask Help: eval('openHelp(312)')
      mask Display: image(imread('Path.png'))
  SELF_Demux : Subsystem  Tag=demux/SelfPort  mask(PreScan Demux Block:){}
      mask help:
      | The SELF port shows (state) information of the actor itself. The outputs are position in the experiment's axis system and the GPS coordinates, and the object's absolute velocity and compass heading.
      |
      | For more information, please click Help.
      settings: DeleteFcn=PreScanBlockDeleteFcn;
      mask Help: eval('openHelp(462)')
      mask Display:
      | port_label('output',1,'x [m]')
      | port_label('output',2,'y [m]')
      | port_label('output',3,'z [m]','texmode','on')
      | port_label('output',4,'Rotx [deg]','texmode','on')
      | port_label('output',5,'Roty [deg]','texmode','on')
      | port_label('output',6,'Rotz [deg]','texmode','on')
      | port_label('output',7,'GPS lat [deg]','texmode','on')
      | port_label('output',8,'GPS long [deg]','texmode','on')
      | port_label('output',9,'GPS alt [m]','texmode','on')
      | port_label('output',10,'Velocity [m/s]')
      | port_label('output',11,'Heading [deg]')
      | port_label('output',12,'Yaw rate [deg/s]')
      | port_label('output',13,'Timestamp [s]')
  STATE_Citroen_C3_Hatchback_1_rc : RateTransition  Tag=mux_rc/StatePort  OutPortSampleTimeOpt=Inherit
  SpeedProfile : S-Function  LoadFcn=load('PrescanMotionData.mat')  FunctionName=sfun_SpeedProfile  Parameters=speedProfileUniqueID, mbxruntime.parameters.convert(timestep)  SFunctionDeploymentMode=off  EnableBusSupport=off  mask(SpeedProfile){speedProfileUniqueID=W01_Base_World_point_cloud_performance_cs_9a6e020116cabe98, timestep=1/20}
      mask prompts: speedProfileUniqueID "Speed Profile Unique ID"; timestep "MATLAB timestep:"
      mask help:
      | The speed profile block outputs the travelled distance, velocities and acceleration along a given path.
      |
      | For more information, please click Help.
      mask Help: eval('openHelp(312)')
      mask Display: image(imread('SpeedProfile.png'))
  Terminator_{1..7} (7 alike) : Terminator
  message_creator : Subsystem
  STATE_Citroen_C3_Hatchback_1_bus : Outport  Tag=outport/StatePort  OutDataTypeStr=Bus: PRESCAN_STATEACTUATORDATA  PortDimensions=1  SampleTime=1/20
  SafetyPlannerLoc : Outport  Port=2
  wires:
  Car_Pos_and_Orient/1(Out1) -> message_creator/1(In1)
  message_creator/1(Out1) -> SafetyPlannerLoc/1
  SELF_Demux/1(x [m]) -> Car_Pos_and_Orient/1(In1)
  SELF_Demux/2(y [m]) -> Car_Pos_and_Orient/2(In2)
  SELF_Demux/3(z [m]) -> Car_Pos_and_Orient/3(In3)
  SELF_Demux/4(rotx [deg]) -> Car_Pos_and_Orient/4(In4)
  SELF_Demux/5(roty [deg]) -> Car_Pos_and_Orient/5(In5)
  SELF_Demux/6(rotz [deg]) -> Car_Pos_and_Orient/6(In6)
  STATE_Citroen_C3_Hatchback_1_rc/1 -> STATE_Citroen_C3_Hatchback_1_bus/1
  SpeedProfile/1 -> Path/1
  Path/1 -> STATE_Citroen_C3_Hatchback_1_rc/1
  SELF_Citroen_C3_Hatchback_1/1 -> SELF_Demux/1(SELF)
  SELF_Demux/7(GPS lat [deg]) -> Terminator_1/1
  SELF_Demux/8(GPS long [deg]) -> Terminator_2/1
  SELF_Demux/9(GPS alt [m]) -> Terminator_3/1
  SELF_Demux/10(velocity [m/s]) -> Terminator_4/1
  SELF_Demux/11(heading [deg]) -> Terminator_5/1
  SELF_Demux/12(yaw rate [deg/s]) -> Terminator_6/1
  SELF_Demux/13(TimeStamp [s]) -> Terminator_7/1

== system W01_Base_World_point_cloud_performance_cs/Controller ==
  Terminator : Terminator
  sfun_Controller : S-Function  FunctionName=sfun_Controller  Parameters=SParameter1, SParameter2, SParameter3, SParameter4, SParameter5, SParameter6, SParameter7, SParameter8, SParameter9, SParameter10, SampleTime  SFunctionDeploymentMode=off  EnableBusSupport=off  mask(Legacy Function){SFunctionSpec=void prescan_outputFcn(void** work1, PRESCAN_CONTROLLERDATA y1[1]), SParameter1=uint8([ExperimentFile 0]), SParameter2=uint8([ModelDepo 0]), SParameter3=uint8([ControllerOptions 0]), SParameter4=RTmode, SParameter5=PreScanExecutionMode, SParameter6=ControlMode, SParameter7=ControllerCount, SParameter8=ControllerIndex, SParameter9=uint8([SimulationMode 0]), SParameter10=uint8([TargetName 0]), SampleTime=TimeStep, ShowSpec=on}
      mask prompts: SParameter1 "P1:"; SParameter2 "P2:"; SParameter3 "P3:"; SParameter4 "P4:"; SParameter5 "P5:"; SParameter6 "P6:"; SParameter7 "P7:"; SParameter8 "P8:"; SParameter9 "P9:"; SParameter10 "P10:"; SampleTime "Sample time (-1 for inherited):"; ShowSpec "Display function specification"
      mask help:
      | This block allows you to call the legacy functions specified by the following Legacy Code Tool definition:
      | def.SFunctionName = 'sfun_Controller';
      | def.OutputFcnSpec = 'void prescan_outputFcn(void** work1, PRESCAN_CONTROLLERDATA y1[1])';
      | def.StartFcnSpec = 'void prescan_startFcn(void ** work1, uint8 p1[], uint8 p2[], uint8 p3[], double p4, double p5, double p6, double p7, double p8, uint8 p9[], uint8 p10[])';
      | def.TerminateFcnSpec = 'void prescan_terminateFcn(void** work1)';
      | def.HeaderFiles = {'prescan_controller_data.h', 'prescan_SFunLibrary.h', 'prescan_CreateLogHandler.h', 'prescan_CreateErrorHandler.h', 'prescan_modify.h', 'ModuleDLL.h'};
      | def.SourceFiles = {'prescan_MexLogHandler.c', 'prescan_SimStructErrorHandler.c', 'prescan_LogHandler.c', 'prescan_ErrorHandler.c', 'prescan_Modify.c'};
      | def.HostLibFiles = {'sensorinterfaced.lib'};
      | def.TargetLibFiles = {'sensorinterfaced.so'};
      | def.IncPaths = {'.', 'C:\projects\prescan\rt_vislibrary\vis\..\pimp\include\sensors\InterfaceRTW'};
      | def.SrcPaths = {'C:\projects\prescan\rt_vislibrary\vis\..\pimp\include\sensors\InterfaceRTW', 'C:\projects\prescan\rt_vislibrary\vis\..\pimp\include\sensors\InterfaceRTW\ccurrt'};
      | def.LibPaths = {'C:\\projects\\prescan\\vislibrary_build\lib'};
      | def.SampleTime = 'parameterized';
      mask Help: <p>This block was generated automatically by the Legacy Code Tool. For detailed help on this tool, call<a href="matlab:legacy_code('help')"> legacy_code('help')</a>.</p>
      mask Callback ShowSpec:
      | if strcmp(get_param(gcbh, 'ShowSpec'), 'on')
      |   set_param(gcbh, 'MaskDisplay', sprintf('fprintf(''%s'');', get_param(gcbh, 'SFunctionSpec')));
      | else
      |   set_param(gcbh, 'MaskDisplay', sprintf('fprintf(''%s'');', get_param(gcbh, 'FunctionName')));
      | end
      mask Display: fprintf('void prescan_outputFcn(void** work1, PRESCAN_CONTROLLERDATA y1[1])');
  wires:
  sfun_Controller/1 -> Terminator/1
